simulink model "MPC"  (R2013b)
settings: Solver=ode45  StartTime=0.0  StopTime=50  RelTol=1e-3
libraries: simulink_extras x4
settings Model: Creator=Maksimus  LastModifiedBy=Maksimus

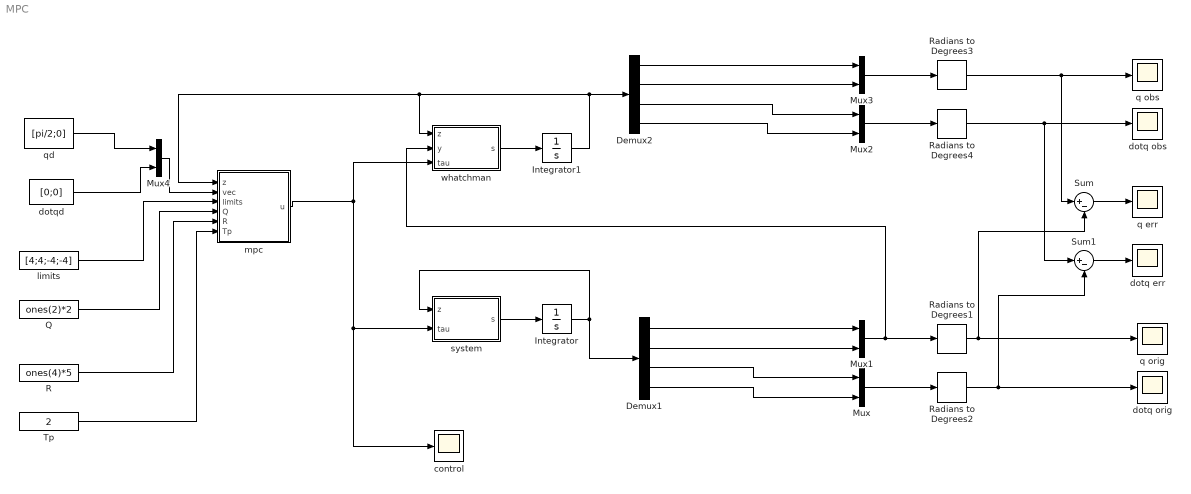
== system MPC ==
  Demux1 : Demux
  Demux2 : Demux
  Integrator : Integrator  InitialCondition=[-pi/2;0;0;0]
  Integrator1 : Integrator  InitialCondition=[-pi/2;0;0;0]
  Mux{,1..4} (5 alike) : Mux  Inputs=2
  Q : Constant  Value=ones(2)*2
  R : Constant  Value=ones(4)*5
  Radians to Degrees{1..4} (4 alike) : simulink_extras/Transformations/Radians to Degrees
  Sum : Sum  Inputs=|+-
  Sum1 : Sum  Inputs=|+-
  Tp : Constant  Value=2
  control : Scope
      settings: YMin=-110  YMax=110  SaveName=ScopeData6
  dotq err : Scope
      settings: YMin=-5.5e+14  YMax=3e+14  SaveName=ScopeData4
  dotq obs : Scope
      settings: YMin=-5.5e+06  YMax=4e+06
  dotq orig : Scope
      settings: YMin=0  YMax=30000  SaveName=ScopeData3
  dotqd : Constant  Value=[0;0]
  limits : Constant  Value=[4;4;-4;-4]
  mpc : MATLAB Function  TreatAsAtomicUnit=on
  q err : Scope
      settings: YMin=-1.4e+06  YMax=500000  SaveName=ScopeData5
  q obs : Scope
  q orig : Scope
      settings: SaveName=ScopeData2
  qd : Constant  Value=[pi/2;0]
  system : MATLAB Function  TreatAsAtomicUnit=on
  whatchman : MATLAB Function  TreatAsAtomicUnit=on
  wires:
  Mux/1 -> Radians to Degrees2/1
  Demux1/1 -> Mux1/1
  Demux1/4 -> Mux/2
  Demux1/3 -> Mux/1
  Radians to Degrees2/1 -> dotq orig/1, Sum1/2
  Demux1/2 -> Mux1/2
  whatchman/1(s) -> Integrator1/1
  Mux2/1 -> Radians to Degrees4/1
  Demux2/1 -> Mux3/1
  Mux3/1 -> Radians to Degrees3/1
  Radians to Degrees3/1 -> q obs/1, Sum/1
  Demux2/4 -> Mux2/2
  Demux2/3 -> Mux2/1
  Demux2/2 -> Mux3/2
  Sum1/1 -> dotq err/1
  Sum/1 -> q err/1
  system/1(s) -> Integrator/1
  Integrator/1 -> Demux1/1, system/1(z)
  Integrator1/1 -> Demux2/1, whatchman/1(z), mpc/1(z)
  mpc/1(u) -> whatchman/3(tau), control/1, system/2(tau)
  Mux1/1 -> whatchman/2(y), Radians to Degrees1/1
  Radians to Degrees4/1 -> Sum1/1, dotq obs/1
  Radians to Degrees1/1 -> Sum/2, q orig/1
  qd/1 -> Mux4/1
  dotqd/1 -> Mux4/2
  Mux4/1 -> mpc/2(vec)
  limits/1 -> mpc/3(limits)
  R/1 -> mpc/5(R)
  Q/1 -> mpc/4(Q)
  Tp/1 -> mpc/6(Tp)

== matlab function MPC/whatchman ==
  data: z input; y input; s output; tau input
function s = fcn(z,y,tau)
%задаем систему
m1 = 1;
m2 = 1;
lc1 = 1;
lc2 = 2;
I1 = 0.12;
I2 = 0.12;
l1 = 1;
l2 = 1;
g=10;
m = [m1;m2];
lc = [lc1;lc2];
I = [I1;I2];
l = [l1;l2];
q =z(1:2);
dotq =z(3:4);

theta = [m(1)*lc(1)^2 + m(2)*l(1)^2 + I(1); m(2) * lc(2)^2 + I(2); m(2)*l(1)*lc(2); m(1)*lc(1) + m(2)*l(1); m(2)*lc(2)]; 

H = [theta(1) + theta(2) + 2 * theta(3)*cos(q(2)), theta(2) + theta(3) * cos(q(2));
    theta(2) + theta(3) * cos(q(2)), theta(2)]; 

C = [-theta(3) * sin(q(2)) * dotq(2), -theta(3) * sin(q(2)) * dotq(2) - theta(3) * sin(q(2)) * dotq(1);
    theta(3) * sin(q(2)) * dotq(1), 0];

G = [ theta(4) * g * cos(q(1)) + theta(5) * g * cos(q(1) + q(2)); theta(5) * g * cos(q(1) + q(2))]; %nonhorizontal robotarm
%конец задания системы
g1=1; %две константы, для того чтобы ошибка убывала
g2 =4;

qcorrection =  g1* (y - q); %поправка для вектора углов
dotqcorrection =  g2*(y -q); %поправка для вектора скоростей
InvH = H^(-1);
InvHC = InvH * C;
InvHG = InvH * G;
tmpsys = - InvHC * dotq - InvHG + InvH*tau;
sys = [dotq + qcorrection ;tmpsys + dotqcorrection ]; 

s = sys;

== matlab function MPC/mpc ==
  data: z input; u output; vec input; limits input; Q input; R input; Tp input
function u = fcn(z,vec,limits, Q, R, Tp)
[x,fval] = fminunc(@(u) J(z,vec,u,2,0.05),repmat([0 0],2/0.05));
u = x(1,:)';

== matlab function MPC/system ==
  data: z input; s output; tau input
function s = fcn(z,tau)
%global linA linB linConst
%s = linA * z + linB * u + linConst;
m1 = 1;
m2 = 1;
lc1 = 1;
lc2 = 2;
I1 = 0.12;
I2 = 0.12;
l1 = 1;
l2 = 1;
g=10;

m = [m1;m2];
lc = [lc1;lc2];
I = [I1;I2];
l = [l1;l2];
dotq = z(3:4);
q = z(1:2);
theta = [m(1)*lc(1)^2 + m(2)*l(1)^2 + I(1); m(2) * lc(2)^2 + I(2); m(2)*l(1)*lc(2); m(1)*lc(1) + m(2)*l(1); m(2)*lc(2)]; 

H = [theta(1) + theta(2) + 2 * theta(3)*cos(q(2)), theta(2) + theta(3) * cos(q(2));
    theta(2) + theta(3) * cos(q(2)), theta(2)]; %is symmetrie, positive definite for all q

%H(q) - 2C(q, dotq) is a skew-syrnmetric matrix

C = [-theta(3) * sin(q(2)) * dotq(2), -theta(3) * sin(q(2)) * dotq(2) - theta(3) * sin(q(2)) * dotq(1);
    theta(3) * sin(q(2)) * dotq(1), 0];

G = [ theta(4) * g * cos(q(1)) + theta(5) * g * cos(q(1) + q(2)); theta(5) * g * cos(q(1) + q(2))]; %nonhorizontal robotarm
%G = [0;0];

InvH = H^(-1);
InvHC = InvH * C;
InvHG = InvH * G;
tmpsys = - InvHC * dotq - InvHG + InvH*tau;
sys = [dotq;tmpsys];

s = sys;
